simulink model "untitled"  (R2023a)
settings: Solver=VariableStepAuto  StartTime=0.0  StopTime=10.0  RelTol=1e-3
settings Model: Creator=a2320606  LastModifiedBy=a2320606

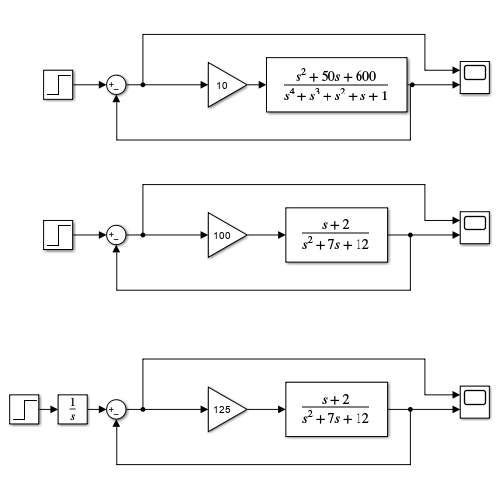
[thumbnail: Simulink's stored preview of the top-level diagram]
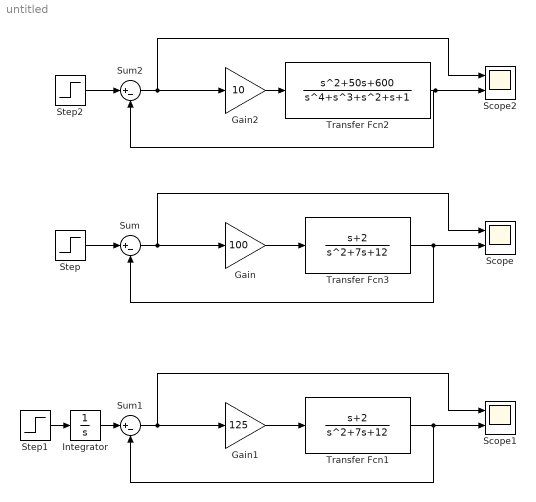
== system untitled ==
  Gain : Gain  Gain=100
  Gain1 : Gain  Gain=125
  Gain2 : Gain  Gain=10
  Integrator : Integrator
  Scope : Scope  NumInputPorts=2
  Scope1 : Scope  NumInputPorts=2
  Scope2 : Scope  NumInputPorts=2
  Step : Step  Time=15  SampleTime=0
  Step1 : Step  Time=15  SampleTime=0
  Step2 : Step  Time=15  SampleTime=0
  Sum : Sum  Inputs=|+-
  Sum1 : Sum  Inputs=|+-
  Sum2 : Sum  Inputs=|+-
  Transfer Fcn1 : TransferFcn  Numerator=[1 2]  Denominator=[1 7 12]
  Transfer Fcn2 : TransferFcn  Numerator=[1 50 600]  Denominator=[1 1 1 1 1]
  Transfer Fcn3 : TransferFcn  Numerator=[1 2]  Denominator=[1 7 12]
  wires:
  Gain/1 -> Transfer Fcn3/1
  Transfer Fcn3/1 -> Sum/2, Scope/2
  Sum/1 -> Gain/1, Scope/1
  Step/1 -> Sum/1
  Sum1/1 -> Gain1/1, Scope1/1
  Gain1/1 -> Transfer Fcn1/1
  Transfer Fcn1/1 -> Sum1/2, Scope1/2
  Step1/1 -> Integrator/1
  Step2/1 -> Sum2/1
  Gain2/1 -> Transfer Fcn2/1
  Sum2/1 -> Gain2/1, Scope2/1
  Transfer Fcn2/1 -> Sum2/2, Scope2/2
  Integrator/1 -> Sum1/1
